simulink model "ROTH_Test"  (R2016a)
settings: Solver=FixedStepDiscrete  StartTime=0.0  StopTime=16  FixedStep=0.005  RelTol=1e-3
undefined symbols (not defined in the file): map, sigbuilder_block
libraries: ROTH x1
settings Model: Creator=oelkawok  LastModifiedBy=oelkawok
settings DataIOCC: SaveOutput=off  SaveTime=off

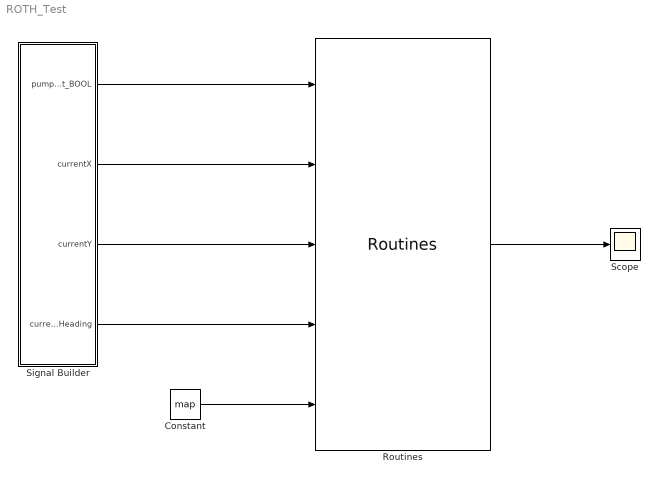
== system ROTH_Test ==
  Constant : Constant  Value=map
  Routines : ROTH/Routines
  Scope : Scope
  Signal Builder : Subsystem  Tag=STV Subsys  LoadFcn=sigbuilder_block('load',[437.4 187.2 550.8 400.2 ]);  StartFcn=sigbuilder_block('start');  StopFcn=sigbuilder_block('stop');  ClipboardFcn=sigbuilder_block('clipboard');  mask(Sigbuilder block){}
      mask help: Simulink:masks:SigbuilderBlock_MD
      mask init:
      | if ~strcmp(get_param(bdroot(gcbh),'SimulationStatus'),'stopped') tuvar = sigbuilder_block('maskInit'); end
      settings: CopyFcn=sigbuilder_block('copy');  DeleteFcn=sigbuilder_block('delete');  ModelCloseFcn=sigbuilder_block('modelClose');  PreSaveFcn=sigbuilder_block('preSave');  PauseFcn=sigbuilder_block('pause');  ContinueFcn=sigbuilder_block('continue');  NameChangeFcn=sigbuilder_block('namechange');  OpenFcn=sigbuilder_block('open',[437.6 199.2 550.4 400 ]);  CloseFcn=sigbuilder_block('close');
      mask Display: plot(0, 0, 100, 100,[2, 2, 32, 32, 2], [68, 8, 8, 68, 68],[32, 2], [38, 38], [32, 19, 2],[53, 60, 44], [32, 17, 17, 2],[16, 16, 31, 31]);txt = getActiveGroup(gcbh);text(2, 100, txt,'verticalAlignment', 'top');
  wires:
  Constant/1 -> Routines/5
  Routines/1 -> Scope/1
  Signal Builder/1(pumperInterrupt_BOOL) -> Routines/1
  Signal Builder/2(currentX) -> Routines/2
  Signal Builder/3(currentY) -> Routines/3
  Signal Builder/4(currentHeading) -> Routines/4

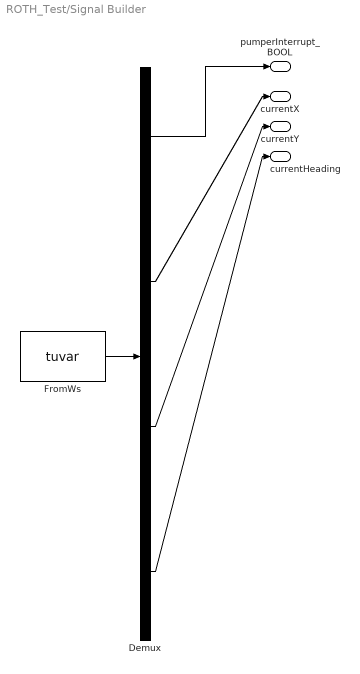
== system ROTH_Test/Signal Builder ==
  Demux : Demux  Tag=STV Demux
  FromWs : FromWorkspace  Tag=STV FromWs  VariableName=tuvar  SampleTime=0
      SigBuilderData=|
      | common.afterFinalStr = 'Extrapolate'
      | common.sampleTime = 0
      | dataSet.timeRange = [0 10]
      | dataSet.name = 'GTSP'
      | sbobj.Groups.Name = 'GTSP'
      | sbobj.Groups.Signals(1).Name = 'pumperInterrupt_BOOL'
      | sbobj.Groups.Signals(1).XData = [0 0.08 0.08 4.74 4.74 4.9 4.9 10]
      | sbobj.Groups.Signals(1).YData = [1 1 0 0 1 1 0 0]
      | sbobj.Groups.Signals(2).Name = 'currentX'
      | sbobj.Groups.Signals(2).XData = [0 2 2 2.58 3.6 5 5 10]
      | sbobj.Groups.Signals(2).YData = [10 10 9 9 9 9 10 10]
      | sbobj.Groups.Signals(3).Name = 'currentY'
      | sbobj.Groups.Signals(3).XData = [0 4 6 6 10]
      | sbobj.Groups.Signals(3).YData = [2 2 2 0 0]
      | sbobj.Groups.Signals(4).Name = 'currentHeading'
      | sbobj.Groups.Signals(4).XData = [0 2 2 5 5 6 6 10]
      | sbobj.Groups.Signals(4).YData = [270 270 180 180 90 90 0 0]
  pumperInterrupt_BOOL : Outport  Tag=STV Outport
  currentX : Outport  Tag=STV Outport  Port=2
  currentY : Outport  Tag=STV Outport  Port=3
  currentHeading : Outport  Tag=STV Outport  Port=4
  wires:
  Demux/1 -> pumperInterrupt_BOOL/1
  FromWs/1 -> Demux/1
  Demux/2 -> currentX/1
  Demux/3 -> currentY/1
  Demux/4 -> currentHeading/1
